simulink model "planmodel2023b"  (R2023b)
settings: Solver=ode4  StartTime=0.0  StopTime=50  FixedStep=0.001  RelTol=1e-3
values from neighbouring files (symbols this model uses):
  a0 = 340.294    [basedata.m]    (also in basedata.mat; control_design.mat; landing_init.m; landing_plan.mat)
  b_ref = 2.0    (= 2)    [basedata.m]    (also in basedata.mat; control_design.mat; landing_init.m; landing_plan.mat)
  c_gear = [0.8e4, 1.4e4, 1.4e4]    [basedata.m]    (also in basedata.mat = [8000 14000 14000]; control_design.mat = [8000 14000 14000]; landing_init.m; landing_plan.mat = [8000 14000 14000])
  c_lat = [1.4e4, 2.2e4, 2.2e4]    [basedata.m]    (also in basedata.mat = [14000 22000 22000]; control_design.mat = [14000 22000 22000]; landing_init.m; landing_plan.mat = [14000 22000 22000])
  c_ref = 0.9    [basedata.m]    (also in basedata.mat; control_design.mat; landing_init.m; landing_plan.mat)
  c_roll = [0.020, 0.018, 0.018]    [basedata.m]    (also in basedata.mat = [0.02 0.018 0.018]; control_design.mat = [0.02 0.018 0.018]; landing_init.m; landing_plan.mat = [0.02 0.018 0.018])
  CD0 = 0.045    [basedata.m]    (also in basedata.mat; canshujisuan.m; control_design.mat; landing_init.m)
  CL0 = 0.083    [basedata.m]    (also in basedata.mat; control_design.mat; landing_init.m; landing_plan.mat)
  CLa = 3.80    (= 3.8)    [basedata.m]    (also in basedata.mat; canshujisuan.m = 2.5; control_design.mat; landing_init.m)
  Clb = -0.08    [basedata.m]    (also in basedata.mat; control_design.mat; landing_init.m; landing_plan.mat)
  Clda = -0.20    (= -0.2)    [basedata.m]    (also in basedata.mat; control_design.mat; landing_init.m; landing_plan.mat)
  CLde = 0.28    [basedata.m]    (also in basedata.mat; control_design.mat; landing_init.m; landing_plan.mat)
  Clp = -0.70    (= -0.7)    [basedata.m]    (also in basedata.mat; control_design.mat; landing_init.m; landing_plan.mat)
  CLq = 4.50    (= 4.5)    [basedata.m]    (also in basedata.mat; canshujisuan.m = 3; control_design.mat; landing_init.m)
  Clr = 0.08    [basedata.m]    (also in basedata.mat; control_design.mat; landing_init.m; landing_plan.mat)
  Cm0 = 0.060    (= 0.06)    [basedata.m]    (also in basedata.mat; control_design.mat; landing_init.m; landing_plan.mat)
  Cma = -0.80    (= -0.8)    [basedata.m]    (also in basedata.mat; control_design.mat; landing_init.m; landing_plan.mat)
  Cmde = -0.90    (= -0.9)    [basedata.m]    (also in basedata.mat; control_design.mat; landing_init.m; landing_plan.mat)
  Cmq = -18.0    (= -18)    [basedata.m]    (also in basedata.mat; control_design.mat; landing_init.m; landing_plan.mat)
  Cnb = 0.25    [basedata.m]    (also in basedata.mat; control_design.mat; landing_init.m; landing_plan.mat)
  Cndr = -0.15    [basedata.m]    (also in basedata.mat; control_design.mat; landing_init.m; landing_plan.mat)
  Cnp = -0.04    [basedata.m]    (also in basedata.mat; control_design.mat; landing_init.m; landing_plan.mat)
  Cnr = -0.45    [basedata.m]    (also in basedata.mat; control_design.mat; landing_init.m; landing_plan.mat)
  CSb = -0.70    (= -0.7)    [basedata.m]    (also in basedata.mat; control_design.mat; landing_init.m; landing_plan.mat)
  CSdr = 0.18    [basedata.m]    (also in basedata.mat; control_design.mat; landing_init.m; landing_plan.mat)
  CSr = 0.12    [basedata.m]    (also in basedata.mat; control_design.mat; landing_init.m; landing_plan.mat)
  D = 0.5 * rho0 * V^2 * S_ref * CD_current    [canshujisuan.m]
  D0 = 1400    [basedata.m]    (also in basedata.mat; control_design.mat = 800; landing.m; landing_init.m)
  da_max = 25    [basedata.m]    (also in basedata.mat; control_design.mat; landing_init.m; landing_plan.mat)
  da_min = -da_max    (= -25)    [basedata.m]    (also in basedata.mat; control_design.mat; landing_init.m; landing_plan.mat)
  de_max = 25    [basedata.m]    (also in basedata.mat; control_design.mat; landing_init.m; landing_plan.mat)
  de_min = -de_max    (= -25)    [basedata.m]    (also in basedata.mat; control_design.mat; landing_init.m; landing_plan.mat)
  DH = pi / 180    (= 0.0174532925199)    [basedata.m]    (also in basedata.mat; control_design.mat; landing_init.m; landing_plan.mat)
  dr_max = 25    [basedata.m]    (also in basedata.mat; control_design.mat; landing_init.m; landing_plan.mat)
  dr_min = -dr_max    (= -25)    [basedata.m]    (also in basedata.mat; control_design.mat; landing_init.m; landing_plan.mat)
  g = 9.80665    [basedata.m]    (also in basedata.mat; canshujisuan.m; control_design.mat; landing_init.m)
  gamma0 = 0.0    (= 0)    [plan.m]    (also in plan.mat)
  ground_y = 0.0    (= 0)    [plan.m]    (also in plan.mat)
  HD = 180 / pi    (= 57.2957795131)    [basedata.m]    (also in basedata.mat; control_design.mat; landing_init.m; landing_plan.mat)
  Ixx = 120.0    (= 120)    [basedata.m]    (also in basedata.mat; control_design.mat; landing_init.m; landing_plan.mat)
  Iyy = 480.0    (= 480)    [basedata.m]    (also in basedata.mat; control_design.mat; landing_init.m; landing_plan.mat)
  Izz = 520.0    (= 520)    [basedata.m]    (also in basedata.mat; control_design.mat; landing_init.m; landing_plan.mat)
  K = 0.12    [basedata.m]    (also in basedata.mat; canshujisuan.m = 0.08; control_design.mat; landing_init.m)
  K_alpha = 7.5375    [basedata.mat]    (also in control_design.m = (((wd_pitch^2)-a24))/(2*kesi_pitch*wd_pitch); control_design.mat; controller.m = 9.375; landingplan.mat)
  k_gear = [1.0e5, 3.0e5, 3.0e5]    [basedata.m]    (also in basedata.mat = [100000 300000 300000]; control_design.mat = [100000 300000 300000]; landing_init.m; landing_plan.mat = [100000 300000 300000])
  k_theta0 = 0.0    (= 0)    [plan.m]    (also in plan.mat)
  Kn_pitch = -0.120095403309    [basedata.mat]    (also in control_design.m = -(2.2*g*(wd_pitch)^2)/(Tr*(((wd_pitch)^2)-a24)*V_control*a34; control_design.mat; controller.m = (2.2*wd^2*g)/(Tr*(wd^2-a24)*V_test*a34); landingplan.mat)
  Kw_pitch = -0.483749055178    [basedata.mat]    (also in control_design.m = -2*kesi_pitch*wd_pitch/a25; control_design.mat; controller.m = -(2*zeta*wd) / a25; landingplan.mat)
  m = 600.0    (= 600)    [basedata.m]    (also in basedata.mat; canshujisuan.m; control_design.mat; landing_init.m)
  mu_brake = [0.0, 0.55, 0.55]    [basedata.m]    (also in basedata.mat = [0 0.55 0.55]; control_design.mat = [0 0.55 0.55]; landing_init.m; landing_plan.mat = [0 0.55 0.55])
  omigax0 = 0    [plan.m]    (also in plan.mat)
  omigay0 = 0    [plan.m]    (also in plan.mat)
  omigaz0 = 0    [plan.m]    (also in plan.mat)
  psi0 = 0    [control_design.mat]    (also in landing.m; landing_init.m; landing_init.mat; landing_plan.mat)
  r_left_b = r_gear_b(:,2)    [basedata.m]    (also in basedata.mat = [-0.333333333333 -0.8 0.65]; control_design.mat = [-0.333333333333 -0.8 0.65]; landing_init.m; landing_plan.mat = [-0.333333333333 -0.8 0.65])
  r_nose_b = r_gear_b(:,1)    [basedata.m]    (also in basedata.mat = [2 0 0.65]; control_design.mat = [2 0 0.65]; landing_init.m; landing_plan.mat = [2 0 0.65])
  r_right_b = r_gear_b(:,3)    [basedata.m]    (also in basedata.mat = [-0.333333333333 0.8 0.65]; control_design.mat = [-0.333333333333 0.8 0.65]; landing_init.m; landing_plan.mat = [-0.333333333333 0.8 0.65])
  rho0 = 1.225    [basedata.m]    (also in basedata.mat; canshujisuan.m; control_design.mat; landing_init.m)
  S_ref = 1.2    [basedata.m]    (also in basedata.mat; canshujisuan.m; control_design.mat; landing_init.m)
  v_eps = 0.20    (= 0.2)    [basedata.m]    (also in basedata.mat; control_design.mat; landing_init.m; landing_plan.mat)
  V_min = 3    [control_design.mat]    (also in landing.m; landing_init.m; landing_plan.mat; landingplan.mat)
  Vx0_b = 0.0    (= 0)    [plan.m]    (also in plan.mat)
  Vy0_b = 0.0    (= 0)    [plan.m]    (also in plan.mat)
  Vz0_b = 0.0    (= 0)    [plan.m]    (also in plan.mat)
  wheel_radius = 0.18    [basedata.m]    (also in basedata.mat; control_design.mat; landing_init.m; landing_plan.mat)
  WOW_on = 0.000    (= 0)    [basedata.m]    (also in basedata.mat; control_design.mat; landing_init.m; landing_plan.mat)
  Xg0 = 0    [control_design.mat]    (also in landing.m = -12000; landing_init.m = -12000; landing_init.mat = -8000; landing_plan.mat = -12000)
  Yg0 = 3    [control_design.mat]    (also in landing.m = 0; landing_init.m = 0; landing_init.mat = 0; landing_plan.mat = 0)
  Zg0 = ground_z - wheel_radius - r_gear_b(3,1) + static_deflection    [basedata.m]    (also in basedata.mat = -0.8215943; control_design.mat = -0.8215943; landing.m = -1000; landing_init.m = -1000)
libraries: matrix_library x18, slpidlib x1
(part 1 of 3)
settings Model: SimulationMode=accelerator  Creator=34355  LastModifiedBy=fjy
settings RTWCC: GPUComputeCapability=5.0
settings ConfigComp: CovBoundaryAbsTol=1.0e-5

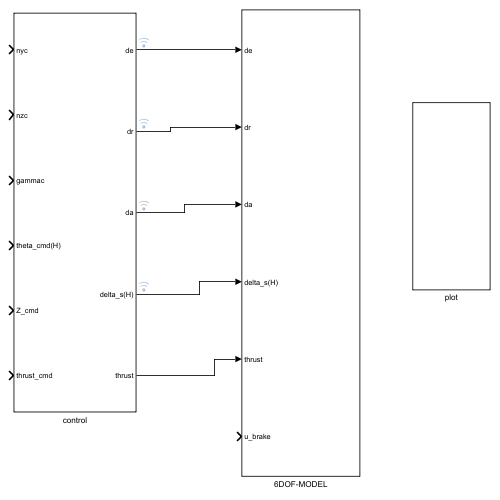
[thumbnail: Simulink's stored preview of the top-level diagram]
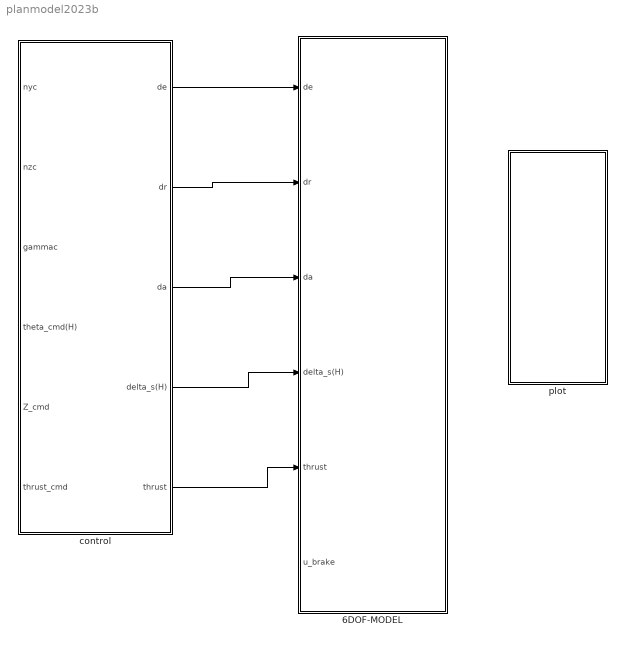
== system planmodel2023b ==
  6DOF-MODEL : Subsystem
  control : Subsystem
  plot : Subsystem
  wires:
  control/1(de) -> 6DOF-MODEL/1(de)
  control/5(thrust) -> 6DOF-MODEL/5(thrust)
  control/4(delta_s(H)) -> 6DOF-MODEL/4(delta_s(H))
  control/2(dr) -> 6DOF-MODEL/2(dr)
  control/3(da) -> 6DOF-MODEL/3(da)

== system planmodel2023b/6DOF-MODEL ==
  de : Inport
  dr : Inport  Port=2
  da : Inport  Port=3
  delta_s(H) : Inport  Port=4
  thrust : Inport  Port=5
  u_brake : Inport  Port=6
  AERO-PARAMETER : Subsystem
  Scope{,1..5} (6 alike) : Scope
  动力学 : Subsystem
  wires:
  动力学/1(alpha(D)) -> Scope/1, AERO-PARAMETER/1(alpha(D))
  thrust/1 -> 动力学/7(thrust)
  u_brake/1 -> 动力学/9(u_brake)
  动力学/2(beta(D)) -> AERO-PARAMETER/2(beta(D))
  动力学/3(wx1) -> AERO-PARAMETER/3(wx1(H))
  动力学/4(wy1) -> AERO-PARAMETER/4(wy1(H))
  动力学/5(wz1) -> AERO-PARAMETER/5(wz1(H))
  de/1 -> AERO-PARAMETER/6(de(D))
  动力学/10(theta(D)) -> Scope1/1
  动力学/6(X) -> Scope2/1
  动力学/7(Y) -> Scope3/1
  动力学/8(Z) -> Scope4/1
  AERO-PARAMETER/1(D) -> 动力学/1(D)
  AERO-PARAMETER/2(L) -> Scope5/1, 动力学/2(L)
  AERO-PARAMETER/3(S) -> 动力学/3(S)
  AERO-PARAMETER/4(MX) -> 动力学/4(MX)
  AERO-PARAMETER/5(MY) -> 动力学/5(MY)
  AERO-PARAMETER/6(MZ) -> 动力学/6(MZ)
  delta_s(H)/1 -> 动力学/8(delta_s(H))
  dr/1 -> AERO-PARAMETER/7(dr(D))
  da/1 -> AERO-PARAMETER/8(da)

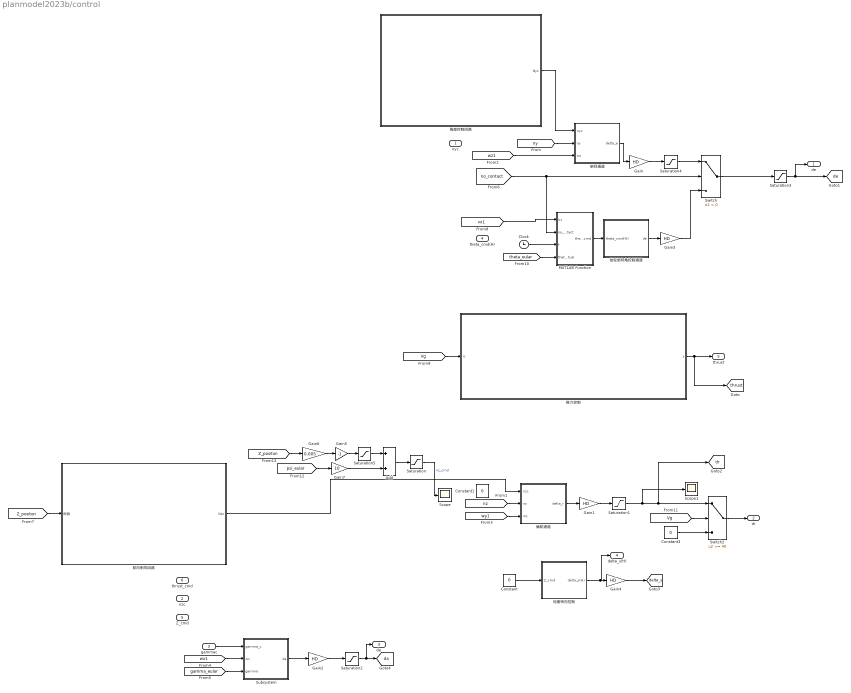
== system planmodel2023b/control ==
  nyc : Inport
  nzc : Inport  Port=2
  gammac : Inport  Port=3
  theta_cmd(H) : Inport  Port=4
  Z_cmd : Inport  Port=5
  thrust_cmd : Inport  Port=6
  Add : Sum
  Clock : Clock
  Constant : Constant  Value=0
  Constant1 : Constant  Value=0
  Constant3 : Constant  Value=0
  Gain{,1..4} (5 alike) : Gain  Gain=HD
  Gain5 : Gain  Gain=-1
  Gain6 : Gain  Gain=0.005
  Gain7 : Gain  Gain=10
  MATLAB Function : MATLAB Function  TreatAsAtomicUnit=on  SystemSampleTime=0.01
  Saturation : Saturate  UpperLimit=2  LowerLimit=-2
  Saturation1 : Saturate  UpperLimit=dr_max  LowerLimit=dr_min
  Saturation2 : Saturate  UpperLimit=da_max  LowerLimit=da_min
  Saturation3 : Saturate  UpperLimit=de_max  LowerLimit=de_min
  Saturation4 : Saturate  UpperLimit=de_max  LowerLimit=de_min
  Saturation5 : Saturate  UpperLimit=0.52  LowerLimit=-0.52
  Scope : Scope
  Scope1 : Scope
  Subsystem : Subsystem
  Switch : Switch  Criteria=u2 > Threshold  SaturateOnIntegerOverflow=off  InputSameDT=off
  Switch2 : Switch  Threshold=40  SaturateOnIntegerOverflow=off  InputSameDT=off
  俯仰通道 : Subsystem
  偏航通道 : Subsystem
  地面转向控制 : Subsystem
  抬轮俯仰角控制通道 : Subsystem
  推力控制 : Subsystem
  航向制导回路 : Subsystem
  高度控制回路 : Subsystem
  de : Outport
  dr : Outport  Port=2
  da : Outport  Port=3
  delta_s(H) : Outport  Port=4
  thrust : Outport  Port=5
  tag scope: da=global, de=global, delta_s=global, dr=global, thrust=global
  wires:
  Gain2/1 -> Saturation2/1
  俯仰通道/1(delta_e) -> Gain/1
  偏航通道/1(delta_r) -> Gain1/1
  Subsystem/1(da) -> Gain2/1
  Saturation2/1 -> [da], da/1
  [wy1] -> 偏航通道/3(wy)
  Saturation1/1 -> Scope1/1, Switch2/1, [dr]
  [wx1] -> Subsystem/2(wx)
  [gamma_eular] -> Subsystem/3(gamma)
  Gain1/1 -> Saturation1/1
  [nz] -> 偏航通道/2(nz)
  抬轮俯仰角控制通道/1(de) -> Gain3/1
  [ny] -> 俯仰通道/2(ny)
  [wz1] -> 俯仰通道/3(wz)
  Gain3/1 -> Switch/3
  gammac/1 -> Subsystem/1(gamma_c)
  Constant/1 -> 地面转向控制/1(Z_cmd)
  Gain4/1 -> [delta_s]
  Gain/1 -> Saturation4/1
  Saturation3/1 -> de/1, [de]
  Clock/1 -> MATLAB Function/3(t)
  MATLAB Function/1(theta_cmd) -> 抬轮俯仰角控制通道/1(theta_cmd(H))
  [vx1] -> MATLAB Function/1(Vx)
  Saturation4/1 -> Switch/1
  Switch/1 -> Saturation3/1
  [no_contact] -> MATLAB Function/2(no_contact), Switch/2
  [Vg] -> 推力控制/1(V)
  推力控制/1(t) -> [thrust], thrust/1
  高度控制回路/1(Nyc) -> 俯仰通道/1(nyc)
  [theta_eular] -> MATLAB Function/4(theta_actual)
  [Vg] -> Switch2/2
  Switch2/1 -> dr/1
  Constant3/1 -> Switch2/3
  地面转向控制/1(delta_s(H)) -> delta_s(H)/1, Gain4/1
  [Z_positon] -> 航向制导回路/1(侧偏)
  Gain5/1 -> Saturation5/1
  Add/1 -> Saturation/1
  [Z_positon] -> Gain6/1
  Gain7/1 -> Add/2
  Gain6/1 -> Gain5/1
  Saturation/1 -> Scope/1  "nz_cmd"
  [psi_eular] -> Gain7/1
  Saturation5/1 -> Add/1
  航向制导回路/1(Nzc) -> 偏航通道/1(nzc)

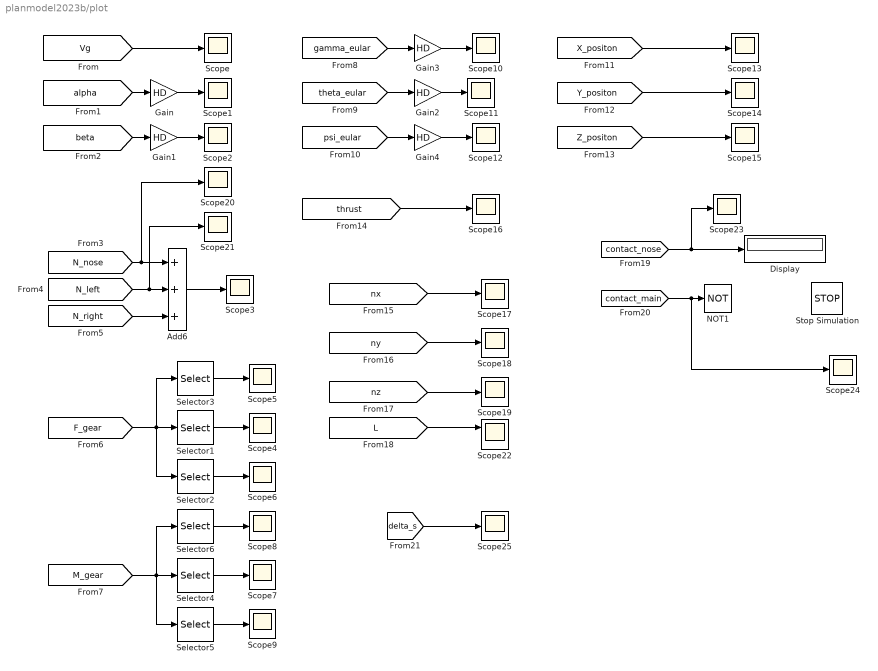
== system planmodel2023b/plot ==
  Add6 : Sum  Inputs=+++
  Display : Display
  Gain{,1..4} (5 alike) : Gain  Gain=HD
  NOT1 : Logic  Operator=NOT  IconShape=distinctive  AllPortsSameDT=off  OutDataTypeStr=boolean
  Scope{,1..21,23..25} (25 alike) : Scope
  Scope22 : Scope  NumInputPorts=2
  Selector1 : Selector  InputPortWidth=3  IndexOptions=Index vector (dialog)  Indices=2  OutputSizes=1
  Selector2 : Selector  InputPortWidth=3  IndexOptions=Index vector (dialog)  Indices=3  OutputSizes=1
  Selector3 : Selector  InputPortWidth=3  IndexOptions=Index vector (dialog)  Indices=1  OutputSizes=1
  Selector4 : Selector  InputPortWidth=3  IndexOptions=Index vector (dialog)  Indices=2  OutputSizes=1
  Selector5 : Selector  InputPortWidth=3  IndexOptions=Index vector (dialog)  Indices=3  OutputSizes=1
  Selector6 : Selector  InputPortWidth=3  IndexOptions=Index vector (dialog)  Indices=1  OutputSizes=1
  Stop Simulation : Stop
  wires:
  [N_nose] -> Add6/1, Scope20/1
  [N_left] -> Add6/2, Scope21/1
  [N_right] -> Add6/3
  [Vg] -> Scope/1
  [alpha] -> Gain/1
  [beta] -> Gain1/1
  Add6/1 -> Scope3/1
  Selector3/1 -> Scope5/1
  Selector2/1 -> Scope6/1
  Selector1/1 -> Scope4/1
  [F_gear] -> Selector2/1, Selector1/1, Selector3/1
  Selector6/1 -> Scope8/1
  Selector4/1 -> Scope7/1
  [M_gear] -> Selector6/1, Selector4/1, Selector5/1
  Selector5/1 -> Scope9/1
  [psi_eular] -> Gain4/1
  [theta_eular] -> Gain2/1
  [gamma_eular] -> Gain3/1
  Gain1/1 -> Scope2/1
  Gain/1 -> Scope1/1
  Gain2/1 -> Scope11/1
  [Y_positon] -> Scope14/1
  [X_positon] -> Scope13/1
  [Z_positon] -> Scope15/1
  Gain3/1 -> Scope10/1
  Gain4/1 -> Scope12/1
  [thrust] -> Scope16/1
  [nx] -> Scope17/1
  [ny] -> Scope18/1
  [nz] -> Scope19/1
  [L] -> Scope22/1
  [contact_nose] -> Display/1, Scope23/1
  [contact_main] -> Scope24/1, NOT1/1
  [delta_s] -> Scope25/1

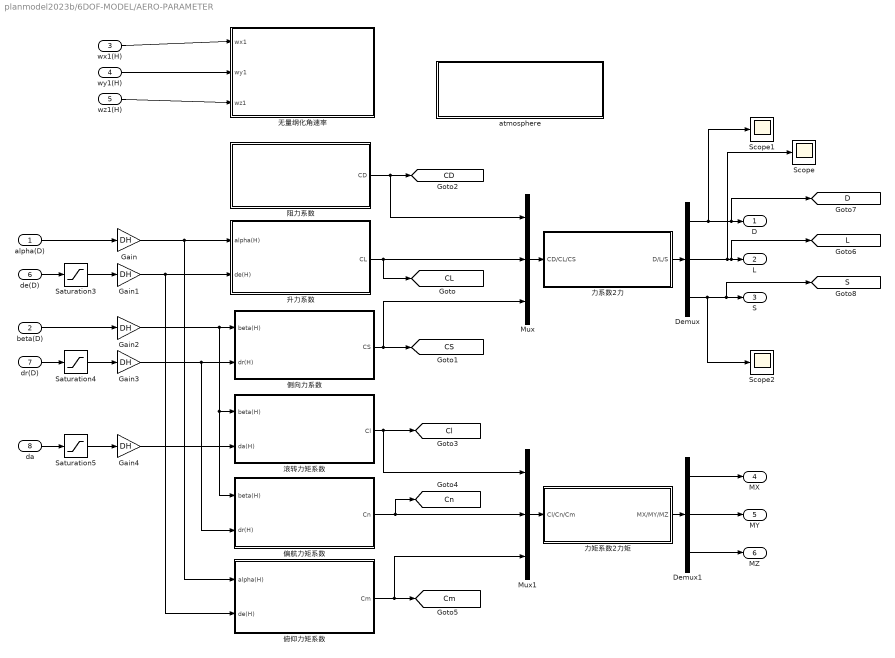
== system planmodel2023b/6DOF-MODEL/AERO-PARAMETER ==
  alpha(D) : Inport
  beta(D) : Inport  Port=2
  wx1(H) : Inport  Port=3
  wy1(H) : Inport  Port=4
  wz1(H) : Inport  Port=5
  de(D) : Inport  Port=6
  dr(D) : Inport  Port=7
  da : Inport  Port=8
  Demux : Demux  Outputs=3
  Demux1 : Demux  Outputs=3
  Gain{,1..4} (5 alike) : Gain  Gain=DH
  Mux : Mux  Inputs=3
  Mux1 : Mux  Inputs=3
  Saturation3 : Saturate  UpperLimit=de_max  LowerLimit=de_min
  Saturation4 : Saturate  UpperLimit=dr_max  LowerLimit=dr_min
  Saturation5 : Saturate  UpperLimit=da_max  LowerLimit=da_min
  Scope : Scope
  Scope1 : Scope
  Scope2 : Scope
  atmosphere : Subsystem
  侧向力系数 : Subsystem
  俯仰力矩系数 : Subsystem
  偏航力矩系数 : Subsystem
  力矩系数2力矩 : Subsystem
  力系数2力 : Subsystem
  升力系数 : Subsystem
  无量纲化角速率 : Subsystem
  滚转力矩系数 : Subsystem
  阻力系数 : Subsystem
  D : Outport
  L : Outport  Port=2
  S : Outport  Port=3
  MX : Outport  Port=4
  MY : Outport  Port=5
  MZ : Outport  Port=6
  tag scope: CD=global, CL=global, CS=global, Cl=global, Cm=global, Cn=global, D=global, L=global, S=global
  wires:
  升力系数/1(CL) -> [CL], Mux/2
  侧向力系数/1(CS) -> Mux/3, [CS]
  da/1 -> Saturation5/1
  Saturation5/1 -> Gain4/1
  Saturation4/1 -> Gain3/1
  dr(D)/1 -> Saturation4/1
  de(D)/1 -> Saturation3/1
  Saturation3/1 -> Gain1/1
  beta(D)/1 -> Gain2/1
  alpha(D)/1 -> Gain/1
  Gain/1 -> 俯仰力矩系数/1(alpha(H)), 升力系数/1(alpha(H))
  Gain1/1 -> 俯仰力矩系数/2(de(H)), 升力系数/2(de(H))
  Gain2/1 -> 侧向力系数/1(beta(H)), 偏航力矩系数/1(beta(H)), 滚转力矩系数/1(beta(H))
  Gain3/1 -> 侧向力系数/2(dr(H)), 偏航力矩系数/2(dr(H))
  Gain4/1 -> 滚转力矩系数/2(da(H))
  wx1(H)/1 -> 无量纲化角速率/1(wx1)
  wy1(H)/1 -> 无量纲化角速率/2(wy1)
  wz1(H)/1 -> 无量纲化角速率/3(wz1)
  阻力系数/1(CD) -> Mux/1, [CD]
  滚转力矩系数/1(Cl) -> [Cl], Mux1/1
  俯仰力矩系数/1(Cm) -> Mux1/3, [Cm]
  偏航力矩系数/1(Cn) -> [Cn], Mux1/2
  Mux/1 -> 力系数2力/1(CD/CL/CS)
  Mux1/1 -> 力矩系数2力矩/1(Cl/Cn/Cm)
  Demux/2 -> Scope/1, [L], L/1
  力系数2力/1(D/L/S) -> Demux/1
  Demux/1 -> Scope1/1, [D], D/1
  Demux/3 -> Scope2/1, [S], S/1
  力矩系数2力矩/1(MX/MY/MZ) -> Demux1/1
  Demux1/1 -> MX/1
  Demux1/2 -> MY/1
  Demux1/3 -> MZ/1

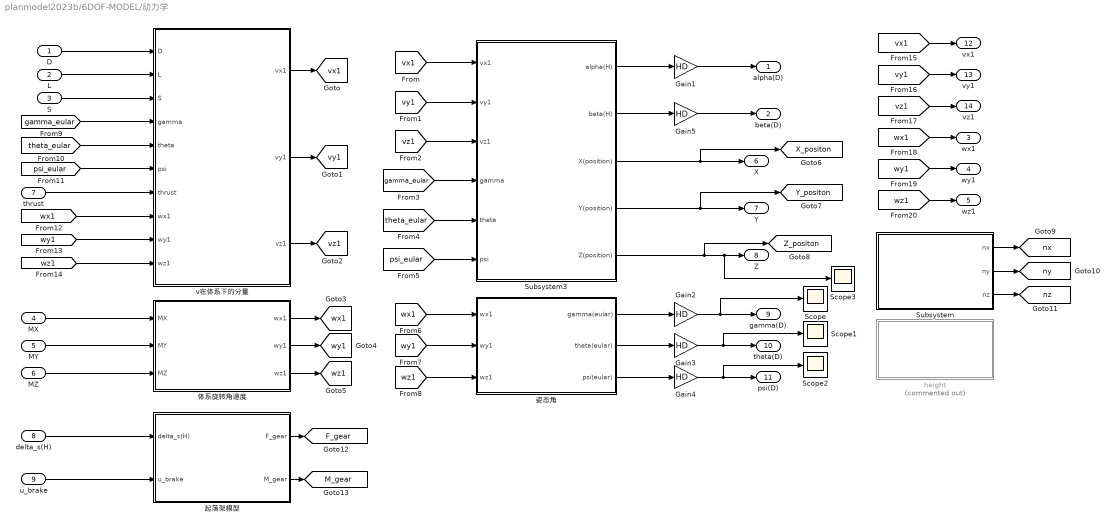
== system planmodel2023b/6DOF-MODEL/动力学 ==
  D : Inport
  L : Inport  Port=2
  S : Inport  Port=3
  MX : Inport  Port=4
  MY : Inport  Port=5
  MZ : Inport  Port=6
  thrust : Inport  Port=7
  delta_s(H) : Inport  Port=8
  u_brake : Inport  Port=9
  Gain{1..5} (5 alike) : Gain  Gain=HD
  Scope{,1..3} (4 alike) : Scope
  Subsystem : Subsystem
  Subsystem3 : Subsystem
  height : Subsystem  Commented=on
  v在体系下的分量 : Subsystem
  体系旋转角速度 : Subsystem
  姿态角 : Subsystem
  起落架模型 : Subsystem
  alpha(D) : Outport
  beta(D) : Outport  Port=2
  wx1 : Outport  Port=3
  wy1 : Outport  Port=4
  wz1 : Outport  Port=5
  X : Outport  Port=6
  Y : Outport  Port=7
  Z : Outport  Port=8
  gamma(D) : Outport  Port=9
  theta(D) : Outport  Port=10
  psi(D) : Outport  Port=11
  vx1 : Outport  Port=12
  vy1 : Outport  Port=13
  vz1 : Outport  Port=14
  tag scope: F_gear=global, M_gear=global, X_positon=global, Y_positon=global, Z_positon=global, nx=global, ny=global, nz=global, vx1=global, vy1=global, vz1=global, wx1=global, wy1=global, wz1=global
  wires:
  MX/1 -> 体系旋转角速度/1(MX)
  MZ/1 -> 体系旋转角速度/3(MZ)
  MY/1 -> 体系旋转角速度/2(MY)
  姿态角/1(gamma(eular)) -> Gain2/1
  姿态角/2(theta(eular)) -> Gain3/1
  姿态角/3(psi(eular)) -> Gain4/1
  thrust/1 -> v在体系下的分量/7(thrust)
  Subsystem3/3(X(position)) -> X/1, [X_positon]
  Subsystem3/4(Y(position)) -> Y/1, [Y_positon]
  Subsystem3/5(Z(position)) -> Scope3/1, Z/1, [Z_positon]
  Gain2/1 -> Scope/1, gamma(D)/1
  Gain3/1 -> theta(D)/1, Scope1/1
  Gain4/1 -> psi(D)/1, Scope2/1
  Subsystem3/2(beta(H)) -> Gain5/1
  Gain5/1 -> beta(D)/1
  Subsystem3/1(alpha(H)) -> Gain1/1
  Gain1/1 -> alpha(D)/1
  v在体系下的分量/1(vx1) -> [vx1]
  v在体系下的分量/2(vy1) -> [vy1]
  v在体系下的分量/3(vz1) -> [vz1]
  体系旋转角速度/3(wz1) -> [wz1]
  体系旋转角速度/2(wy1) -> [wy1]
  体系旋转角速度/1(wx1) -> [wx1]
  [vx1] -> Subsystem3/1(vx1)
  [vy1] -> Subsystem3/2(vy1)
  [vz1] -> Subsystem3/3(vz1)
  [gamma_eular] -> Subsystem3/4(gamma)
  [theta_eular] -> Subsystem3/5(theta)
  [psi_eular] -> Subsystem3/6(psi)
  [wx1] -> 姿态角/1(wx1)
  [wy1] -> 姿态角/2(wy1)
  [wz1] -> 姿态角/3(wz1)
  [gamma_eular] -> v在体系下的分量/4(gamma)
  [theta_eular] -> v在体系下的分量/5(theta)
  [psi_eular] -> v在体系下的分量/6(psi)
  [wx1] -> v在体系下的分量/8(wx1)
  [wy1] -> v在体系下的分量/9(wy1)
  [wz1] -> v在体系下的分量/10(wz1)
  [vx1] -> vx1/1
  [vy1] -> vy1/1
  [vz1] -> vz1/1
  [wx1] -> wx1/1
  [wy1] -> wy1/1
  [wz1] -> wz1/1
  Subsystem/1(nx) -> [nx]
  Subsystem/2(ny) -> [ny]
  Subsystem/3(nz) -> [nz]
  D/1 -> v在体系下的分量/1(D)
  L/1 -> v在体系下的分量/2(L)
  S/1 -> v在体系下的分量/3(S)
  起落架模型/1(F_gear) -> [F_gear]
  起落架模型/2(M_gear) -> [M_gear]
  delta_s(H)/1 -> 起落架模型/1(delta_s(H))
  u_brake/1 -> 起落架模型/2(u_brake)

== system planmodel2023b/control/Subsystem ==
  gamma_c : Inport
  wx : Inport  Port=2
  gamma : Inport  Port=3
  Constant : Constant  Value=0
  Gain1 : Gain  Gain=1/HD
  Integrator : Integrator
  Product : Product
  Product1 : Product
  Product2 : Product
  Scope : Scope  NumInputPorts=2
  Sum : Sum  Inputs=|+-
  Sum1 : Sum  Inputs=|+-
  Sum2 : Sum  Inputs=|++
  kgamma_to_wx : Constant  Value=3
  kigamma_to_wx : Constant  Value=0.8
  kwx_to_da : Constant  Value=0.35
  da : Outport
  wires:
  Sum/1 -> Product/2, Product2/2
  Sum1/1 -> Product1/2
  Product1/1 -> da/1
  wx/1 -> Sum1/2
  gamma/1 -> Scope/2, Sum/2
  kigamma_to_wx/1 -> Product2/1
  Product2/1 -> Integrator/1
  Product/1 -> Sum2/1
  Sum2/1 -> Sum1/1
  Integrator/1 -> Sum2/2
  Gain1/1 -> Scope/1, Sum/1
  kgamma_to_wx/1 -> Product/1
  kwx_to_da/1 -> Product1/1
  Constant/1 -> Gain1/1

== system planmodel2023b/control/俯仰通道 ==
  nyc : Inport
  ny : Inport  Port=2
  wz : Inport  Port=3
  Constant : Constant
  Gain : Gain
  Gain2 : Gain
  Integrator : Integrator  ExternalReset=level  LimitOutput=on  UpperSaturationLimit=5  LowerSaturationLimit=-5
  Ka : Constant  Value=K_alpha
  Kn : Constant  Value=Kn_pitch
  Kwz : Constant  Value=Kw_pitch
  Product : Product
  Product1 : Product
  Product2 : Product
  Scope : Scope  NumInputPorts=2
  Sum{,1..3} (4 alike) : Sum  Inputs=|+-
  伪攻角回路 : Subsystem
  delta_e : Outport
  wires:
  ny/1 -> Scope/2, Sum/2
  nyc/1 -> Scope/1, Sum/1
  Sum/1 -> Product/2
  Product/1 -> Integrator/1
  Integrator/1 -> Sum1/1
  Sum1/1 -> Product1/2
  Product1/1 -> Sum2/1
  Sum2/1 -> Product2/2
  Product2/1 -> delta_e/1
  wz/1 -> 伪攻角回路/1(wz), Sum2/2
  伪攻角回路/1(alpha_c) -> Sum1/2
  Constant/1 -> Sum3/1
  [no_contact] -> Sum3/2
  Sum3/1 -> Integrator/2
  Ka/1 -> Gain/1
  Gain/1 -> Product1/1
  Kn/1 -> Product/1
  Kwz/1 -> Gain2/1
  Gain2/1 -> Product2/1

== system planmodel2023b/control/偏航通道 ==
  nzc : Inport
  nz : Inport  Port=2
  wy : Inport  Port=3
  Constant1 : Constant
  Constant3 : Constant  Value=0
  Gain : Gain  Gain=-0.92
  Gain1 : Gain  Gain=6.68
  Gain2 : Gain  Gain=0.99
  Gain4 : Gain  Gain=HD
  Integrator : Integrator
  Saturation1 : Saturate  UpperLimit=0.2*57.3  LowerLimit=-0.2*57.3
  Scope : Scope  NumInputPorts=2
  Scope1 : Scope
  Scope12 : Scope
  Scope2 : Scope  NumInputPorts=2
  Sum : Sum  Inputs=|+-
  Sum1 : Sum  Inputs=|+-
  Sum2 : Sum  Inputs=|+-
  Switch2 : Switch  Threshold=40  SaturateOnIntegerOverflow=off  InputSameDT=off
  伪攻角回路 : Subsystem
  delta_r : Outport
  wires:
  nz/1 -> Scope/2, Sum/2
  nzc/1 -> Scope/1, Sum/1
  Constant1/1 -> Switch2/1
  Constant3/1 -> Switch2/3
  [Vg] -> Switch2/2
  Gain4/1 -> Scope12/1
  [psi_eular] -> Gain4/1
  wy/1 -> Scope2/2, Sum2/2, 伪攻角回路/1(wy)
  伪攻角回路/1(beta_c) -> Sum1/2
  Sum1/1 -> Gain1/1
  Gain1/1 -> Scope2/1, Sum2/1
  Sum2/1 -> Gain2/1
  Gain2/1 -> Scope1/1, delta_r/1
  Gain/1 -> Integrator/1
  Sum/1 -> Gain/1
  Integrator/1 -> Saturation1/1
  Saturation1/1 -> Sum1/1

== system planmodel2023b/control/地面转向控制 ==
  Z_cmd : Inport
  Constant2 : Constant  Value=0
  Gain : Gain  Gain=0.8
  Gain4 : Gain  Gain=HD
  K_r : Constant
  K_z : Constant  Value=0.05
  Product : Product
  Product2 : Product
  Scope : Scope  NumInputPorts=2
  Scope12 : Scope
  Scope25 : Scope
  Step : Step  After=5*pi/180  SampleTime=0
  Sum : Sum  Inputs=|+-
  Sum1 : Sum  Inputs=|++
  Sum2 : Sum  Inputs=|++
  Switch1 : Switch  Criteria=u2 > Threshold  Threshold=40  SaturateOnIntegerOverflow=off  InputSameDT=off
  delta_s(H) : Outport
  wires:
  Z_cmd/1 -> Scope/1, Sum/1
  [Z_positon] -> Scope/2, Sum/2
  K_z/1 -> Product/1
  Sum1/1 -> Sum2/1
  [wz1] -> Product2/1
  K_r/1 -> Product2/2
  [delta_s] -> Scope25/1
  [psi_eular] -> Gain/1
  Gain4/1 -> Scope12/1
  [psi_eular] -> Gain4/1
  Product2/1 -> Sum2/2
  Gain/1 -> Sum1/2
  Sum/1 -> Product/2
  [Vg] -> Switch1/2
  Constant2/1 -> Switch1/1
  Sum2/1 -> Switch1/3
  Switch1/1 -> delta_s(H)/1
  Product/1 -> Sum1/1

== system planmodel2023b/control/抬轮俯仰角控制通道 ==
  theta_cmd(H) : Inport
  Gain1 : Gain
  K_theta : Gain  Gain=1.3
  Sum : Sum  Inputs=|+-
  Sum1 : Sum  Inputs=|+-
  de : Outport
  wires:
  theta_cmd(H)/1 -> Sum/1
  [theta_eular] -> Sum/2
  Sum/1 -> K_theta/1
  K_theta/1 -> Sum1/1
  Sum1/1 -> de/1
  [wz1] -> Gain1/1
  Gain1/1 -> Sum1/2

== system planmodel2023b/control/推力控制 ==
  V : Inport
  Constant : Constant  Value=200
  Constant1 : Constant  Value=3000
  Constant2 : Constant  Value=200
  Gain : Gain
  PID Controller2 : slpidlib/PID Controller  Controller=PID  Form=Parallel  TimeDomain=Continuous-time  UseExternalTs=off  SampleTime=-1  IntegratorMethod=Forward Euler  FilterMethod=Forward Euler  ControllerParametersSource=internal  P=0.5  I=0  UseKiTs=off  D=0.3  N=0  UseFilter=on  TunerSelectOption=Transfer Function Based (PID Tuner App)  InitialConditionSource=internal  InitialConditionForIntegrator=0  InitialConditionForFilter=0  DifferentiatorICPrevScaledInput=0  ExternalReset=none  TrackingMode=off  Kt=1  LimitOutput=on  SatLimitsSource=internal  UpperSaturationLimit=1  LowerSaturationLimit=0  LinearizeAsGain=on  AntiWindupMode=clamping  Kb=1  LimitIntegrator=off  UpperIntegratorSaturationLimit=inf  LowerIntegratorSaturationLimit=-inf  POutMin=[]  POutMax=[]  IOutMin=[]  IOutMax=[]  DOutMin=[]  DOutMax=[]  NOutMin=[]  NOutMax=[]  SumOutMin=[]  SumOutMax=[]  SaturationOutMin=[]  SaturationOutMax=[]  PParamMin=[]  PParamMax=[]  IParamMin=[]  IParamMax=[]  DParamMin=[]  DParamMax=[]  NParamMin=[]  NParamMax=[]  KbParamMin=[]  KbParamMax=[]  KtParamMin=[]  KtParamMax=[]  KbOutMin=[]  KbOutMax=[]  KtOutMin=[]  KtOutMax=[]  IntegratorOutMin=[]  IntegratorOutMax=[]  FilterOutMin=[]  FilterOutMax=[]  SumI1OutMin=[]  SumI1OutMax=[]  SumI2OutMin=[]  SumI2OutMax=[]  SumI3OutMin=[]  SumI3OutMax=[]  SumI4OutMin=[]  SumI4OutMax=[]  SumDOutMin=[]  SumDOutMax=[]  DifferentiatorOutMin=[]  DifferentiatorOutMax=[]  FilterDiffOutCoefMin=[]  FilterDiffOutCoefMax=[]  ReciprocalOutMin=[]  ReciprocalOutMax=[]  SumDenOutMin=[]  SumDenOutMax=[]  SumNumOutMin=[]  SumNumOutMax=[]  DivideOutMin=[]  DivideOutMax=[]  UdiffTsProdOutMin=[]  UdiffTsProdOutMax=[]  NTsProdOutMin=[]  NTsProdOutMax=[]  UintegralTsProdOutMin=[]  UintegralTsProdOutMax=[]  UngainTsProdOutMin=[]  UngainTsProdOutMax=[]  ClampingZeroOutDataTypeStr=Inherit: Inherit via back propagation  ClampingZeroOutMin=[]  ClampingZeroOutMax=[]  FilterDenConstantOutDataTypeStr=Inherit: Inherit via back propagation  FilterDenConstantOutMin=[]  FilterDenConstantOutMax=[]  PCopyOutDataTypeStr=Inherit: Inherit via back propagation  PCopyOutMin=[]  PCopyOutMax=[]  NCopyOutDataTypeStr=Inherit: Inherit via back propagation  NCopyOutMin=[]  NCopyOutMax=[]  IntegratorContinuousStateAttributes=''  IntegratorStateMustResolveToSignalObject=off  IntegratorRTWStateStorageClass=Auto  FilterContinuousStateAttributes=''  FilterStateMustResolveToSignalObject=off  FilterRTWStateStorageClass=Auto  ParallelPVariant=InternalParameters  IdealPVariant=Disabled  IVariant=InternalParameters  DVariant=InternalParameters  IntegratorVariant=Continuous  SatVariant=Enabled  AWVariant=ContClampingParallel  PCopyVariant=Disabled  TRVariant=Disabled  FdbkBlocksVariant=Forward  IdealPFdbkVariant=Disabled  SatFdbkVariant=Disabled  DerivativeFilterVariant=ContFilter  NVariant=InternalParameters  NCopyVariant=Disabled  FilterICVariant=InternalICsFilter  IntegratorICVariant=InternalICs  ExternalResetVariant=Disabled  TRSumVariant=Passthrough  SumFdbkVariant=Disabled  SumVariant=Sum_PID  TsampFilterVariant=InternalTs  TsampNgainVariant=Passthrough  TsampIntegralVariant=Disabled_SignalSpec  ExternalSaturationOutDataTypeStr=Inherit: Same as second input
  Product : Product
  Sum : Sum  Inputs=|+-
  Switch : Switch  Criteria=u2 > Threshold  Threshold=1000  SaturateOnIntegerOverflow=off  InputSameDT=off
  t : Outport
  tag scope: t=global
  wires:
  Constant1/1 -> Product/1
  Product/1 -> t/1, [t]
  V/1 -> Sum/2
  PID Controller2/1 -> Gain/1
  Sum/1 -> PID Controller2/1
  Gain/1 -> Product/2
  Switch/1 -> Sum/1
  Constant/1 -> Switch/1
  [Y_positon] -> Switch/2
  Constant2/1 -> Switch/3

== system planmodel2023b/control/航向制导回路 ==
  侧偏 : Inport
  Abs1 : Abs  SaturateOnIntegerOverflow=off
  Abs3 : Abs  SaturateOnIntegerOverflow=off
  Constant : Constant  Value=0
  Constant3 : Constant  Value=1.8
  MinMax : MinMax  Inputs=2
  Product2 : Product
  Scope2 : Scope  NumInputPorts=2
  Scope5 : Scope
  Scope8 : Scope
  Selector : Selector  InputPortWidth=3  IndexOptions=Index vector (dialog)  Indices=[3]  OutputSizes=1
  Sign : Signum
  Sum3 : Sum  Inputs=|+-
  Sum4 : Sum  Inputs=|+-
  kdy : Gain  Gain=-0.2
  kdy_dot : Gain  Gain=0.5
  Nzc : Outport
  wires:
  侧偏/1 -> Scope2/2, Sum3/2
  Constant/1 -> Scope2/1, Sum3/1
  Sum3/1 -> kdy/1
  Abs1/1 -> MinMax/1
  Sign/1 -> Product2/1
  Constant3/1 -> Abs3/1
  MinMax/1 -> Product2/2
  Abs3/1 -> MinMax/2
  Product2/1 -> Scope5/1, Nzc/1
  Sum4/1 -> kdy_dot/1
  kdy_dot/1 -> Abs1/1, Sign/1, Scope8/1
  kdy/1 -> Sum4/1
  Selector/1 -> Sum4/2
  [V_ground] -> Selector/1

== system planmodel2023b/control/高度控制回路 ==
  Abs1 : Abs  SaturateOnIntegerOverflow=off
  Constant : Constant  Value=1000
  Constant1 : Constant
  Constant2 : Constant  Value=3
  Divide : Product  Inputs=*/
  Gain1 : Gain
  MinMax : MinMax  Inputs=2
  Product : Product
  Product2 : Product
  Saturation : Saturate  UpperLimit=35  LowerLimit=-35
  Saturation1 : Saturate  UpperLimit=10  LowerLimit=-10
  Scope1 : Scope  NumInputPorts=2
  Scope4 : Scope
  Selector : Selector  InputPortWidth=3  IndexOptions=Index vector (dialog)  Indices=[2]  OutputSizes=1
  Sign : Signum
  Sum : Sum  Inputs=-+
  Sum1 : Sum  Inputs=|+-
  Sum2 : Sum
  Trigonometric Function : Trigonometry  Operator=cos
  Trigonometric Function1 : Trigonometry  Operator=cos
  kh : Gain  Gain=0.04
  khd : Gain  Gain=0.15
  Nyc : Outport
  wires:
  Gain1/1 -> Abs1/1, Sign/1
  kh/1 -> Sum1/1
  [Y_positon] -> Sum/1, Scope1/1
  khd/1 -> Sum1/2
  Sum2/1 -> Gain1/1
  Sign/1 -> Product2/1
  Sum1/1 -> Sum2/2
  Constant2/1 -> MinMax/2
  MinMax/1 -> Product2/2
  [theta_eular] -> Trigonometric Function/1
  Product2/1 -> Nyc/1, Scope4/1
  Abs1/1 -> MinMax/1
  Constant/1 -> Scope1/2, Sum/2
  [V_ground] -> Selector/1
  [gamma_eular] -> Trigonometric Function1/1
  Trigonometric Function1/1 -> Product/1
  Trigonometric Function/1 -> Product/2
  Product/1 -> Divide/2
  Constant1/1 -> Divide/1
  Divide/1 -> Sum2/1
  Saturation1/1 -> khd/1
  Saturation/1 -> kh/1
  Sum/1 -> Saturation/1
  Selector/1 -> Saturation1/1

== system planmodel2023b/6DOF-MODEL/AERO-PARAMETER/atmosphere ==
  Constant : Constant  Value=0
  Constant1 : Constant  Value=rho0
  Constant2 : Constant  Value=a0
  Constant3 : Constant  Value=0.5
  Display : Display
  Product : Product  Inputs=3
  Square : Math  Operator=square
  Subtract : Sum  Inputs=+-
  tag scope: Va=global, Vwind=global, a_sound=global, qc=global, rho=global
  wires:
  [Vg] -> Subtract/1
  [Vwind] -> Subtract/2
  Subtract/1 -> [Va]
  Constant/1 -> [Vwind]
  Constant1/1 -> [rho]
  Constant2/1 -> [a_sound]
  Constant3/1 -> Product/1
  [rho] -> Product/2
  Product/1 -> Display/1, [qc]
  Square/1 -> Product/3
  [Va] -> Square/1

== system planmodel2023b/6DOF-MODEL/AERO-PARAMETER/侧向力系数 ==
  beta(H) : Inport
  dr(H) : Inport  Port=2
  Add : Sum  Inputs=+++
  Constant1 : Constant  Value=CSb
  Constant2 : Constant  Value=CSr
  Constant3 : Constant  Value=CSdr
  Product : Product
  Product2 : Product
  Product3 : Product
  CS : Outport
  wires:
  Add/1 -> CS/1
  Constant3/1 -> Product2/2
  Product2/1 -> Add/3
  dr(H)/1 -> Product2/1
  beta(H)/1 -> Product/1
  Constant1/1 -> Product/2
  Constant2/1 -> Product3/2
  [r_hat] -> Product3/1
  Product/1 -> Add/1
  Product3/1 -> Add/2

== system planmodel2023b/6DOF-MODEL/AERO-PARAMETER/俯仰力矩系数 ==
  alpha(H) : Inport
  de(H) : Inport  Port=2
  Add : Sum  Inputs=++++
  Constant : Constant  Value=Cm0
  Constant1 : Constant  Value=Cma
  Constant2 : Constant  Value=Cmq
  Constant3 : Constant  Value=Cmde
  Product : Product
  Product2 : Product
  Product3 : Product
  Cm : Outport
  wires:
  Product2/1 -> Add/4
  de(H)/1 -> Product2/1
  Constant3/1 -> Product2/2
  alpha(H)/1 -> Product/1
  Constant1/1 -> Product/2
  Add/1 -> Cm/1
  Constant2/1 -> Product3/2
  [q_hat] -> Product3/1
  Product3/1 -> Add/3
  Product/1 -> Add/2
  Constant/1 -> Add/1

== system planmodel2023b/6DOF-MODEL/AERO-PARAMETER/偏航力矩系数 ==
  beta(H) : Inport
  dr(H) : Inport  Port=2
  Add : Sum  Inputs=++++
  Constant1 : Constant  Value=Cnb
  Constant2 : Constant  Value=Cnp
  Constant3 : Constant  Value=Cndr
  Constant4 : Constant  Value=Cnr
  Product{,1..3} (4 alike) : Product
  Cn : Outport
  wires:
  Product2/1 -> Add/4
  Constant4/1 -> Product1/2
  Product/1 -> Add/1
  dr(H)/1 -> Product2/1
  Constant3/1 -> Product2/2
  beta(H)/1 -> Product/1
  Constant1/1 -> Product/2
  Add/1 -> Cn/1
  Constant2/1 -> Product3/2
  [p_hat] -> Product3/1
  Product1/1 -> Add/3
  [r_hat] -> Product1/1
  Product3/1 -> Add/2

== system planmodel2023b/6DOF-MODEL/AERO-PARAMETER/力矩系数2力矩 ==
  Cl/Cn/Cm : Inport
  Constant : Constant  Value=S_ref
  Constant1 : Constant  Value=c_ref
  Constant2 : Constant  Value=b_ref
  Demux : Demux  Outputs=3
  Mux : Mux  Inputs=3
  Product : Product  Inputs=4
  Product1 : Product  Inputs=4
  Product2 : Product  Inputs=4
  Scope : Scope
  MX/MY/MZ : Outport
  wires:
  Cl/Cn/Cm/1 -> Demux/1
  Demux/1 -> Product/1
  Constant/1 -> Product2/2, Product1/2, Product/2
  Demux/3 -> Product2/1
  Demux/2 -> Product1/1
  [qc] -> Product2/3, Product1/3, Product/3
  Product/1 -> Scope/1, Mux/1
  Product1/1 -> Mux/2
  Product2/1 -> Mux/3
  Mux/1 -> MX/MY/MZ/1
  Constant2/1 -> Product1/4, Product/4
  Constant1/1 -> Product2/4

== system planmodel2023b/6DOF-MODEL/AERO-PARAMETER/力系数2力 ==
  CD/CL/CS : Inport
  Constant : Constant  Value=S_ref
  Demux : Demux  Outputs=3
  Display : Display
  Display1 : Display
  Display2 : Display
  Mux : Mux  Inputs=3
  Product : Product  Inputs=3
  Product1 : Product  Inputs=3
  Product2 : Product  Inputs=3
  D/L/S : Outport
  wires:
  CD/CL/CS/1 -> Demux/1
  Demux/1 -> Product/1
  Constant/1 -> Product2/2, Product1/2, Product/2
  Demux/3 -> Product2/1
  Demux/2 -> Product1/1
  [qc] -> Product2/3, Product1/3, Product/3
  Product/1 -> Display/1, Mux/1
  Product1/1 -> Display1/1, Mux/2
  Product2/1 -> Display2/1, Mux/3
  Mux/1 -> D/L/S/1

== system planmodel2023b/6DOF-MODEL/AERO-PARAMETER/升力系数 ==
  alpha(H) : Inport
  de(H) : Inport  Port=2
  Add : Sum  Inputs=++++
  Constant : Constant  Value=CL0
  Constant1 : Constant  Value=CLa
  Constant2 : Constant  Value=CLq
  Constant3 : Constant  Value=CLde
  Product : Product
  Product2 : Product
  Product3 : Product
  CL : Outport
  wires:
  Constant/1 -> Add/1
  alpha(H)/1 -> Product/1
  Constant1/1 -> Product/2
  Product/1 -> Add/2
  [q_hat] -> Product3/1
  Constant2/1 -> Product3/2
  de(H)/1 -> Product2/1
  Constant3/1 -> Product2/2
  Product2/1 -> Add/4
  Product3/1 -> Add/3
  Add/1 -> CL/1

== system planmodel2023b/6DOF-MODEL/AERO-PARAMETER/无量纲化角速率 ==
  wx1 : Inport
  wy1 : Inport  Port=2
  wz1 : Inport  Port=3
  Constant : Constant  Value=V_min
  Max : MinMax  Function=max  Inputs=2
  Scope : Scope
  Subsystem : Subsystem
  Subsystem1 : Subsystem
  Subsystem2 : Subsystem
  tag scope: Va_safe=global, p_hat=global, q_hat=global, r_hat=global
  wires:
  wx1/1 -> Subsystem2/1(wx1)
  wy1/1 -> Subsystem/1(wy1)
  wz1/1 -> Subsystem1/1(wz1)
  [Va_safe] -> Subsystem2/2(Va), Subsystem1/2(Va), Subsystem/2(Va)
  Subsystem/1(r_hat) -> [r_hat]
  Subsystem1/1(q_hat) -> Scope/1, [q_hat]
  Subsystem2/1(p_hat) -> [p_hat]
  [Va] -> Max/2
  Constant/1 -> Max/1
  Max/1 -> [Va_safe]

== system planmodel2023b/6DOF-MODEL/AERO-PARAMETER/滚转力矩系数 ==
  beta(H) : Inport
  da(H) : Inport  Port=2
  Add : Sum  Inputs=++++
  Constant1 : Constant  Value=Clb
  Constant2 : Constant  Value=Clp
  Constant3 : Constant  Value=Clda
  Constant4 : Constant  Value=Clr
  Product{,1..3} (4 alike) : Product
  Scope{,1..3} (4 alike) : Scope
  Cl : Outport
  wires:
  Product3/1 -> Add/2, Scope1/1
  da(H)/1 -> Product2/1
  Product/1 -> Scope/1, Add/1
  beta(H)/1 -> Product/1
  Add/1 -> Cl/1
  Constant1/1 -> Product/2
  Constant3/1 -> Product2/2
  Constant2/1 -> Product3/2
  [p_hat] -> Product3/1
  Product1/1 -> Scope2/1, Add/3
  [r_hat] -> Product1/1
  Constant4/1 -> Product1/2
  Product2/1 -> Scope3/1, Add/4

== system planmodel2023b/6DOF-MODEL/AERO-PARAMETER/阻力系数 ==
  Add : Sum
  Constant : Constant  Value=CD0
  Constant1 : Constant  Value=K
  Product : Product
  Square : Math  Operator=square
  CD : Outport
  wires:
  Constant/1 -> Add/1
  Constant1/1 -> Product/1
  [CL] -> Square/1
  Square/1 -> Product/2
  Product/1 -> Add/2
  Add/1 -> CD/1

== system planmodel2023b/6DOF-MODEL/动力学/Subsystem ==
  Add : Sum
  Constant : Constant  Value=0
  Constant1 : Constant  Value=0
  Constant2 : Constant  Value=m*g
  Demux : Demux  Outputs=3
  Divide : Product  Inputs=*/
  Mux1 : Mux  Inputs=3
  Mux2 : Mux  Inputs=3
  Reshape1 : Reshape  OutputDimensionality=Column vector (2-D)
  Scope : Scope
  Scope1 : Scope
  nx : Outport
  ny : Outport  Port=2
  nz : Outport  Port=3
  wires:
  Demux/2 -> Scope/1, ny/1
  Add/1 -> Reshape1/1
  [Y1] -> Mux1/2
  [X1] -> Mux1/1
  [Z1] -> Mux1/3
  Constant1/1 -> Mux2/3
  Constant/1 -> Mux2/2
  Mux1/1 -> Add/1
  Mux2/1 -> Add/2
  Reshape1/1 -> Divide/1
  Divide/1 -> Demux/1
  Demux/1 -> nx/1
  Demux/3 -> Scope1/1, nz/1
  [thrust] -> Mux2/1
  Constant2/1 -> Divide/2

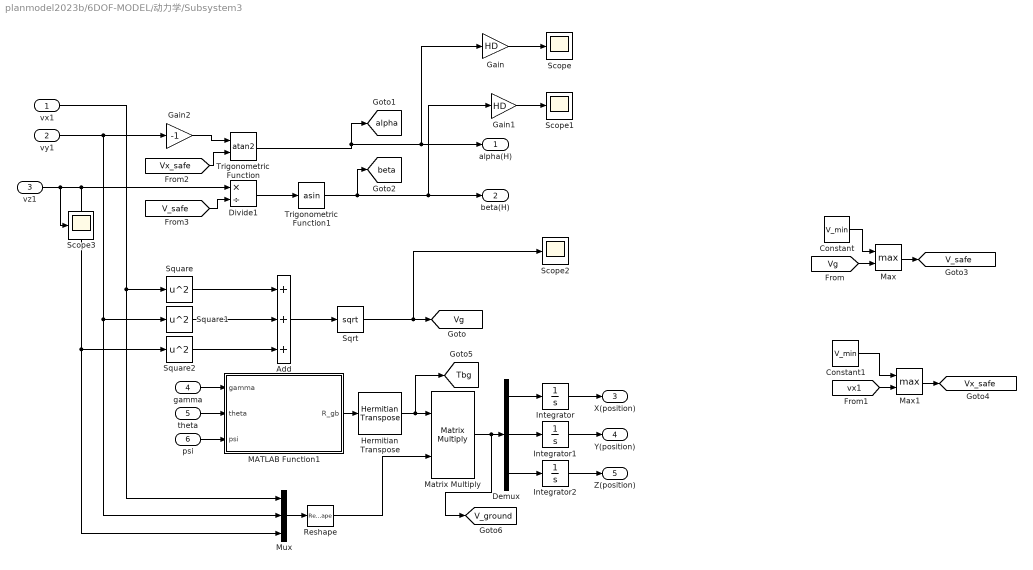
== system planmodel2023b/6DOF-MODEL/动力学/Subsystem3 ==
  vx1 : Inport
  vy1 : Inport  Port=2
  vz1 : Inport  Port=3
  gamma : Inport  Port=4
  theta : Inport  Port=5
  psi : Inport  Port=6
  Add : Sum  Inputs=+++
  Constant : Constant  Value=V_min
  Constant1 : Constant  Value=V_min  VectorParams1D=off
  Demux : Demux  Outputs=3
  Divide1 : Product  Inputs=*/
  Gain : Gain  Gain=HD
  Gain1 : Gain  Gain=HD
  Gain2 : Gain  Gain=-1
  Hermitian Transpose : matrix_library/Hermitian Transpose
      settings: LibrarySourceBlock=|
      | simulink/Matrix
      | Operations/Hermitian Transpose
  Integrator : Integrator  InitialCondition=Xg0
  Integrator1 : Integrator  InitialCondition=Yg0
  Integrator2 : Integrator  InitialCondition=Zg0
  MATLAB Function1 : MATLAB Function  TreatAsAtomicUnit=on
  Matrix Multiply : Product  Multiplication=Matrix(*)
  Max : MinMax  Function=max  Inputs=2
  Max1 : MinMax  Function=max  Inputs=2
  Mux : Mux  Inputs=3
  Reshape : Reshape  OutputDimensionality=Column vector (2-D)
  Scope{,1..3} (4 alike) : Scope
  Sqrt : Sqrt
  Square : Math  Operator=square
  Square1 : Math  Operator=square
  Square2 : Math  Operator=square
  Trigonometric Function : Trigonometry  Operator=atan2
  Trigonometric Function1 : Trigonometry  Operator=asin
  alpha(H) : Outport
  beta(H) : Outport  Port=2
  X(position) : Outport  Port=3
  Y(position) : Outport  Port=4
  Z(position) : Outport  Port=5
  tag scope: Tbg=global, V_ground=global, V_safe=global, Vg=global, Vx_safe=global, alpha=global, beta=global
  wires:
  vy1/1 -> Mux/2, Square1/1, Gain2/1
  Trigonometric Function/1 -> alpha(H)/1, Gain/1, [alpha]
  Mux/1 -> Reshape/1
  Add/1 -> Sqrt/1
  Divide1/1 -> Trigonometric Function1/1
  Trigonometric Function1/1 -> beta(H)/1, Gain1/1, [beta]
  gamma/1 -> MATLAB Function1/1(gamma)
  theta/1 -> MATLAB Function1/2(theta)
  psi/1 -> MATLAB Function1/3(psi)
  MATLAB Function1/1(R_gb) -> Hermitian Transpose/1
  Hermitian Transpose/1 -> [Tbg], Matrix Multiply/1
  Reshape/1 -> Matrix Multiply/2
  Matrix Multiply/1 -> [V_ground], Demux/1
  Demux/1 -> Integrator/1
  Demux/2 -> Integrator1/1
  Demux/3 -> Integrator2/1
  Integrator/1 -> X(position)/1
  Integrator1/1 -> Y(position)/1
  Integrator2/1 -> Z(position)/1
  Gain/1 -> Scope/1
  Gain1/1 -> Scope1/1
  vz1/1 -> Scope3/1, Divide1/1, Mux/3, Square2/1
  vx1/1 -> Square/1, Mux/1
  Square/1 -> Add/1
  Square1/1 -> Add/2
  Square2/1 -> Add/3
  Sqrt/1 -> Scope2/1, [Vg]
  Constant/1 -> Max/1
  Max/1 -> [V_safe]
  [Vg] -> Max/2
  [vx1] -> Max1/2
  Constant1/1 -> Max1/1
  Max1/1 -> [Vx_safe]
  [Vx_safe] -> Trigonometric Function/2
  [V_safe] -> Divide1/2
  Gain2/1 -> Trigonometric Function/1

== system planmodel2023b/6DOF-MODEL/动力学/height ==
  Constant : Constant  Commented=on  Value=0
  Constant1 : Constant  Commented=on  Value=0
  Constant2 : Constant  Commented=on
  Demux1 : Demux  Commented=on  Outputs=3
  From : From  Commented=on  GotoTag=height  TagVisibility=global
  From1 : From  Commented=on  GotoTag=Y_positon  TagVisibility=global
  From11 : From  Commented=on  GotoTag=az1  TagVisibility=global
  From12 : From  Commented=on  GotoTag=gamma_eular  TagVisibility=global
  From13 : From  Commented=on  GotoTag=theta_eular  TagVisibility=global
  From5 : From  Commented=on  GotoTag=psi_eular  TagVisibility=global
  From6 : From  Commented=on  GotoTag=ax1  TagVisibility=global
  From7 : From  Commented=on  GotoTag=ay1  TagVisibility=global
  Goto : Goto  Commented=on  GotoTag=height  TagVisibility=global
  Goto4 : Goto  Commented=on  GotoTag=axg  TagVisibility=global
  Goto5 : Goto  Commented=on  GotoTag=ayg  TagVisibility=global
  Goto6 : Goto  Commented=on  GotoTag=azg  TagVisibility=global
  Hermitian Transpose1 : matrix_library/Hermitian Transpose  Commented=on
  MATLAB Function2 : MATLAB Function  Commented=on  TreatAsAtomicUnit=on
  Matrix Multiply1 : Product  Commented=on  Multiplication=Matrix(*)
  Mux1 : Mux  Commented=on  Inputs=3
  Scope : Scope  Commented=on
  Stop Simulation : Stop  Commented=on
  Switch : Switch  Commented=on  Criteria=u2 > Threshold  SaturateOnIntegerOverflow=off  InputSameDT=off
  Switch1 : Switch  Commented=on  Criteria=u2 > Threshold  SaturateOnIntegerOverflow=off  InputSameDT=off
  To Workspace : ToWorkspace  Commented=on  VariableName=H_OUT  SaveFormat=Timeseries  SampleTime=-1
  wires:
  From1/1 -> Switch/2, Switch/1
  Constant/1 -> Switch/3
  Switch/1 -> To Workspace/1, Goto/1, Scope/1
  From6/1 -> Mux1/1
  From13/1 -> MATLAB Function2/2(theta)
  MATLAB Function2/1(R_gb) -> Hermitian Transpose1/1
  From5/1 -> MATLAB Function2/3(psi)
  From7/1 -> Mux1/2
  Mux1/1 -> Matrix Multiply1/2
  From12/1 -> MATLAB Function2/1(gamma)
  Matrix Multiply1/1 -> Demux1/1
  From11/1 -> Mux1/3
  Demux1/3 -> Goto6/1
  Demux1/1 -> Goto4/1
  Demux1/2 -> Goto5/1
  Hermitian Transpose1/1 -> Matrix Multiply1/1
  Switch1/1 -> Stop Simulation/1
  From/1 -> Switch1/2
  Constant1/1 -> Switch1/1
  Constant2/1 -> Switch1/3

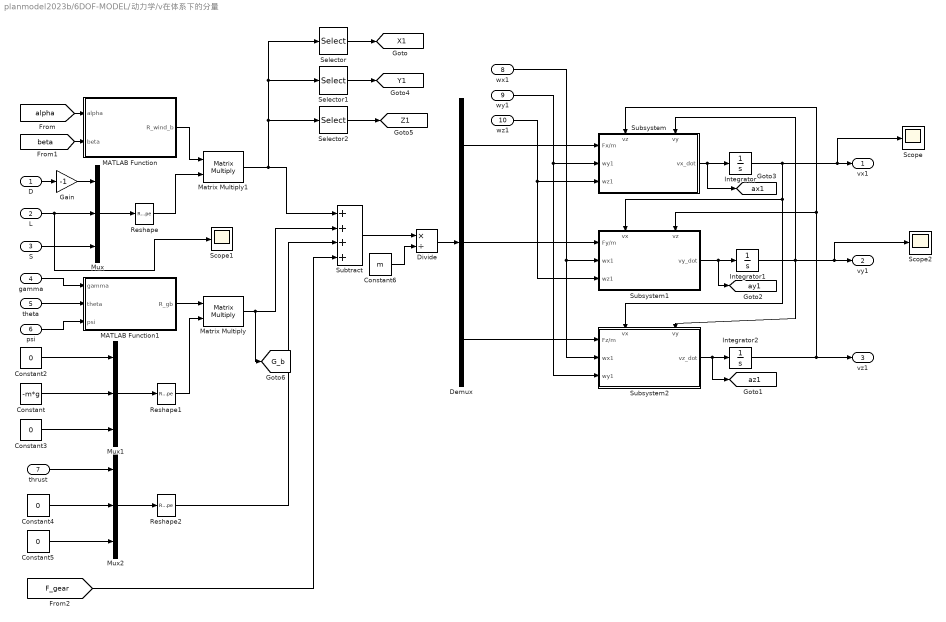
== system planmodel2023b/6DOF-MODEL/动力学/v在体系下的分量 ==
  D : Inport
  L : Inport  Port=2
  S : Inport  Port=3
  gamma : Inport  Port=4
  theta : Inport  Port=5
  psi : Inport  Port=6
  thrust : Inport  Port=7
  wx1 : Inport  Port=8
  wy1 : Inport  Port=9
  wz1 : Inport  Port=10
  Constant : Constant  Value=-m*g
  Constant{2..5} (4 alike) : Constant  Value=0
  Constant6 : Constant  Value=m
  Demux : Demux  Outputs=3
  Divide : Product  Inputs=*/
  Gain : Gain  Gain=-1
  Integrator : Integrator  InitialCondition=Vx0_b
  Integrator1 : Integrator  InitialCondition=Vy0_b
  Integrator2 : Integrator  InitialCondition=Vz0_b
  MATLAB Function : MATLAB Function  TreatAsAtomicUnit=on
  MATLAB Function1 : MATLAB Function  TreatAsAtomicUnit=on
  Matrix Multiply : Product  Multiplication=Matrix(*)
  Matrix Multiply1 : Product  Multiplication=Matrix(*)
  Mux : Mux  Inputs=3
  Mux1 : Mux  Inputs=3
  Mux2 : Mux  Inputs=3
  Reshape : Reshape  OutputDimensionality=Column vector (2-D)
  Reshape1 : Reshape  OutputDimensionality=Column vector (2-D)
  Reshape2 : Reshape  OutputDimensionality=Column vector (2-D)
  Scope : Scope
  Scope1 : Scope
  Scope2 : Scope
  Selector : Selector  InputPortWidth=3  IndexOptions=Index vector (dialog)  Indices=1  OutputSizes=1
  Selector1 : Selector  InputPortWidth=3  IndexOptions=Index vector (dialog)  Indices=2  OutputSizes=1
  Selector2 : Selector  InputPortWidth=3  IndexOptions=Index vector (dialog)  Indices=3  OutputSizes=1
  Subsystem : Subsystem
      settings: PortSchema="{\"entries\":[{\"content\":{\"sides\":[{\"content\":{\"connectorIds\":[\"In1\",\"In2\",\"In3\"]},\"type\":\"ConnectorPlacement.EquallySpacedRectSide\",\"uuid\":\"7ff87203-b960-4b2e-98b2-52440802f400\"},{\"content\":{\"connectorIds\":[\"Out1\"],\"side\":\"RIGHT\"},\"type\":\"ConnectorPlacement.EquallySpacedRectSide\",\"uuid\":\"9c9feb08-84fd-4a54-9043-b4ead2e4096f\"},{\"content\":{\"connectorIds\":[\"In4\",\"In5\"],\"side\":\"TOP\"},\"type\":\"ConnectorPlacement.EquallySpacedRectSide\",\"uuid\":\"1cdec289-1739-4022-8a1c-b747968e9695\"}]},\"type\":\"ConnectorPlacement.EquallySpacedConnector\",\"uuid\":\"02dfab66-3ffd-47f9-ab8e-2ebbe405c5eb\"}],\"packageUris\":[\"http://schema.mathworks.com/mf0/Connector/R2020b\"],\"version\":\"1.0\"}"
  Subsystem1 : Subsystem
      settings: PortSchema="{\"entries\":[{\"content\":{\"sides\":[{\"content\":{\"connectorIds\":[\"In1\",\"In2\",\"In3\"]},\"type\":\"ConnectorPlacement.EquallySpacedRectSide\",\"uuid\":\"7ff87203-b960-4b2e-98b2-52440802f400\"},{\"content\":{\"connectorIds\":[\"Out1\"],\"side\":\"RIGHT\"},\"type\":\"ConnectorPlacement.EquallySpacedRectSide\",\"uuid\":\"9c9feb08-84fd-4a54-9043-b4ead2e4096f\"},{\"content\":{\"connectorIds\":[\"In4\",\"In5\"],\"side\":\"TOP\"},\"type\":\"ConnectorPlacement.EquallySpacedRectSide\",\"uuid\":\"1cdec289-1739-4022-8a1c-b747968e9695\"}]},\"type\":\"ConnectorPlacement.EquallySpacedConnector\",\"uuid\":\"02dfab66-3ffd-47f9-ab8e-2ebbe405c5eb\"}],\"packageUris\":[\"http://schema.mathworks.com/mf0/Connector/R2020b\"],\"version\":\"1.0\"}"
  Subsystem2 : Subsystem
      settings: PortSchema="{\"entries\":[{\"content\":{\"sides\":[{\"content\":{\"connectorIds\":[\"In1\",\"In2\",\"In3\"]},\"type\":\"ConnectorPlacement.EquallySpacedRectSide\",\"uuid\":\"7ff87203-b960-4b2e-98b2-52440802f400\"},{\"content\":{\"connectorIds\":[\"Out1\"],\"side\":\"RIGHT\"},\"type\":\"ConnectorPlacement.EquallySpacedRectSide\",\"uuid\":\"9c9feb08-84fd-4a54-9043-b4ead2e4096f\"},{\"content\":{\"connectorIds\":[\"In4\",\"In5\"],\"side\":\"TOP\"},\"type\":\"ConnectorPlacement.EquallySpacedRectSide\",\"uuid\":\"1cdec289-1739-4022-8a1c-b747968e9695\"}]},\"type\":\"ConnectorPlacement.EquallySpacedConnector\",\"uuid\":\"02dfab66-3ffd-47f9-ab8e-2ebbe405c5eb\"}],\"packageUris\":[\"http://schema.mathworks.com/mf0/Connector/R2020b\"],\"version\":\"1.0\"}"
  Subtract : Sum  Inputs=++++
  vx1 : Outport
  vy1 : Outport  Port=2
  vz1 : Outport  Port=3
  tag scope: G_b=global, X1=global, Y1=global, Z1=global, ax1=global, ay1=global, az1=global
  wires:
  D/1 -> Gain/1
  L/1 -> Scope1/1, Mux/2
  S/1 -> Mux/3
  Mux/1 -> Reshape/1
  Constant2/1 -> Mux1/1
  Constant3/1 -> Mux1/3
  Mux1/1 -> Reshape1/1
  Constant4/1 -> Mux2/2
  Constant5/1 -> Mux2/3
  gamma/1 -> MATLAB Function1/1(gamma)
  theta/1 -> MATLAB Function1/2(theta)
  psi/1 -> MATLAB Function1/3(psi)
  MATLAB Function1/1(R_gb) -> Matrix Multiply/1
  Reshape1/1 -> Matrix Multiply/2
  Matrix Multiply/1 -> [G_b], Subtract/2
  Subtract/1 -> Divide/1
  Divide/1 -> Demux/1
  Constant6/1 -> Divide/2
  Integrator/1 -> Scope/1, vx1/1, Subsystem1/4(vx), Subsystem2/4(vx)
  Integrator1/1 -> Scope2/1, vy1/1, Subsystem/5(vy), Subsystem2/5(vy)
  Integrator2/1 -> vz1/1, Subsystem1/5(vz), Subsystem/4(vz)
  Demux/1 -> Subsystem/1(Fx/m)
  wz1/1 -> Subsystem/3(wz1), Subsystem1/3(wz1)
  wy1/1 -> Subsystem2/3(wy1), Subsystem/2(wy1)
  Demux/2 -> Subsystem1/1(Fy/m)
  Subsystem1/1(vy_dot) -> [ay1], Integrator1/1
  Subsystem/1(vx_dot) -> [ax1], Integrator/1
  Demux/3 -> Subsystem2/1(Fz/m)
  Subsystem2/1(vz_dot) -> [az1], Integrator2/1
  wx1/1 -> Subsystem1/2(wx1), Subsystem2/2(wx1)
  Mux2/1 -> Reshape2/1
  Reshape2/1 -> Subtract/3
  Constant/1 -> Mux1/2
  thrust/1 -> Mux2/1
  MATLAB Function/1(R_wind_b) -> Matrix Multiply1/1
  Reshape/1 -> Matrix Multiply1/2
  Matrix Multiply1/1 -> Selector1/1, Selector/1, Selector2/1, Subtract/1
  [alpha] -> MATLAB Function/1(alpha)
  [beta] -> MATLAB Function/2(beta)
  [F_gear] -> Subtract/4
  Selector2/1 -> [Z1]
  Selector1/1 -> [Y1]
  Selector/1 -> [X1]
  Gain/1 -> Mux/1

== system planmodel2023b/6DOF-MODEL/动力学/体系旋转角速度 ==
  MX : Inport
  MY : Inport  Port=2
  MZ : Inport  Port=3
  Add : Sum
  Add1 : Sum
  Add2 : Sum
  Demux : Demux  Outputs=3
  MATLAB Function : MATLAB Function  TreatAsAtomicUnit=on
  Matrix Multiply1 : Product  Multiplication=Matrix(*)
  Mux : Mux  Inputs=3
  Selector : Selector  InputPortWidth=3  IndexOptions=Index vector (dialog)  Indices=1  OutputSizes=1
  Selector1 : Selector  InputPortWidth=3  IndexOptions=Index vector (dialog)  Indices=2  OutputSizes=1
  Selector2 : Selector  InputPortWidth=3  IndexOptions=Index vector (dialog)  Indices=3  OutputSizes=1
  Subsystem : Subsystem
  Subsystem1 : Subsystem
  Subsystem2 : Subsystem
  wx1 : Outport
  wy1 : Outport  Port=2
  wz1 : Outport  Port=3
  wires:
  Subsystem/1(wx1) -> Subsystem2/2(wx1), Subsystem1/2(wx1), wx1/1
  Subsystem1/1(wy1) -> wy1/1, Subsystem2/3(wy1), Subsystem/3(wy1)
  Subsystem2/1(wz1) -> wz1/1, Subsystem1/3(wz1), Subsystem/2(wz1)
  [M_gear] -> Selector2/1, Selector1/1, Selector/1
  MX/1 -> Add/1
  MY/1 -> Add1/1
  MZ/1 -> Add2/1
  Selector/1 -> Add/2
  Selector2/1 -> Add2/2
  Selector1/1 -> Add1/2
  MATLAB Function/1(R_wind_b) -> Matrix Multiply1/1
  [alpha] -> MATLAB Function/1(alpha)
  [beta] -> MATLAB Function/2(beta)
  Add/1 -> Mux/1
  Add1/1 -> Mux/2
  Add2/1 -> Mux/3
  Mux/1 -> Matrix Multiply1/2
  Demux/1 -> Subsystem/1(MX)
  Matrix Multiply1/1 -> Demux/1
  Demux/2 -> Subsystem1/1(MY)
  Demux/3 -> Subsystem2/1(MZ)

== system planmodel2023b/6DOF-MODEL/动力学/姿态角 ==
  wx1 : Inport
  wy1 : Inport  Port=2
  wz1 : Inport  Port=3
  Subsystem : Subsystem
  Subsystem1 : Subsystem
  Subsystem2 : Subsystem
  gamma(eular) : Outport
  theta(eular) : Outport  Port=2
  psi(eular) : Outport  Port=3
  tag scope: gamma_eular=global, psi_eular=global, theta_eular=global
  wires:
  wy1/1 -> Subsystem/2(wy1), Subsystem1/1(wy1), Subsystem2/1(wy1)
  wx1/1 -> Subsystem/1(wx1)
  Subsystem/1(gamma(eular)) -> [gamma_eular], gamma(eular)/1
  wz1/1 -> Subsystem1/2(wz1), Subsystem/3(wz1), Subsystem2/2(wz1)
  Subsystem1/1(theta(eular)) -> [theta_eular], theta(eular)/1
  Subsystem2/1(psi(eular)) -> psi(eular)/1, [psi_eular]
